simulink model "term"  (R2019b)
settings: Solver=VariableStepAuto  StartTime=0.0  StopTime=10  RelTol=1e-3
InitFcn:
  | clear all
  | given
values from neighbouring files (symbols this model uses):
  a0 = 0.01    [given.m]
  a1 = 1    [given.m]
  a2 = 1000    [given.m]
  a3 = 1000    [given.m]
  a4 = 10    [given.m]
  alpha = 0.9    [given.m]
  bar_B = [ ... (first row only)    [given.m]
  g = 9.81    [given.m]
  K = [-100 -100 -100 -10]    [given.m]
  kappa = 5    [given.m]
  N = 100    [given.m]
  psi0 = 0    [given.m]
  r0 = 5    [given.m]
  r1 = 10    [given.m]
  theta0 = 0    [given.m]
  x0 = 0    [given.m]
  y0 = 0    [given.m]
  z0 = 0    [given.m]
settings Model: Creator=bedla  LastModifiedBy=bedla

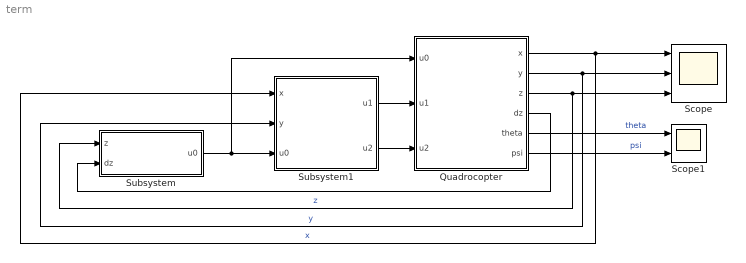
== system term ==
  Quadrocopter : Subsystem
  Scope : Scope  NumInputPorts=3
  Scope1 : Scope  NumInputPorts=2
  Subsystem : Subsystem
  Subsystem1 : Subsystem
  wires:
  Quadrocopter/3(z) -> Subsystem/1(z), Scope/3  "z"
  Subsystem1/1(u1) -> Quadrocopter/2(u1)
  Subsystem1/2(u2) -> Quadrocopter/3(u2)
  Quadrocopter/1(x) -> Subsystem1/1(x), Scope/1  "x"
  Quadrocopter/2(y) -> Subsystem1/2(y), Scope/2  "y"
  Quadrocopter/5(theta) -> Scope1/1  "theta"
  Quadrocopter/6(psi) -> Scope1/2  "psi"
  Subsystem/1(u0) -> Quadrocopter/1(u0), Subsystem1/3(u0)
  Quadrocopter/4(dz) -> Subsystem/2(dz)

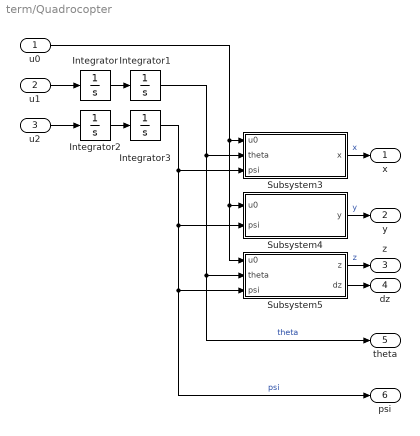
== system term/Quadrocopter ==
  u0 : Inport
  u1 : Inport  Port=2
  u2 : Inport  Port=3
  Integrator : Integrator
  Integrator1 : Integrator  InitialCondition=theta0
  Integrator2 : Integrator
  Integrator3 : Integrator  InitialCondition=psi0
  Subsystem3 : Subsystem
  Subsystem4 : Subsystem
  Subsystem5 : Subsystem
  x : Outport
  y : Outport  Port=2
  z : Outport  Port=3
  dz : Outport  Port=4
  theta : Outport  Port=5
  psi : Outport  Port=6
  wires:
  Integrator3/1 -> Subsystem3/3(psi), Subsystem4/2(psi), psi/1, Subsystem5/3(psi)  "psi"
  Integrator1/1 -> Subsystem3/2(theta), theta/1, Subsystem5/2(theta)  "theta"
  u0/1 -> Subsystem3/1(u0), Subsystem4/1(u0), Subsystem5/1(u0)
  Subsystem3/1(x) -> x/1  "x"
  Subsystem4/1(y) -> y/1  "y"
  Subsystem5/1(z) -> z/1  "z"
  Subsystem5/2(dz) -> dz/1
  u1/1 -> Integrator/1
  u2/1 -> Integrator2/1
  Integrator/1 -> Integrator1/1
  Integrator2/1 -> Integrator3/1

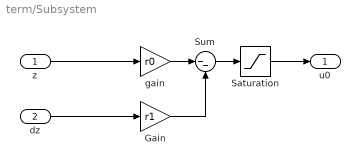
== system term/Subsystem ==
  z : Inport
  dz : Inport  Port=2
  Gain : Gain  Gain=r1
  Saturation : Saturate  UpperLimit=alpha*g  LowerLimit=-alpha*g
  Sum : Sum  Inputs=|--
  gain : Gain  Gain=r0
  u0 : Outport
  wires:
  Gain/1 -> Sum/2
  Saturation/1 -> u0/1
  z/1 -> gain/1
  gain/1 -> Sum/1
  dz/1 -> Gain/1
  Sum/1 -> Saturation/1

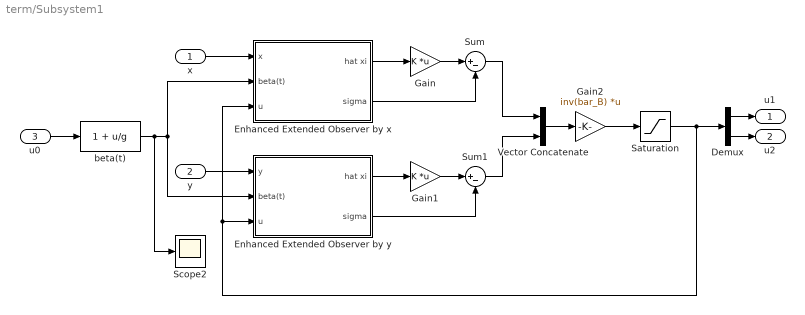
== system term/Subsystem1 ==
  x : Inport
  y : Inport  Port=2
  u0 : Inport  Port=3
  Demux : Demux  Outputs=2
  Enhanced Extended Observer by x : Subsystem
  Enhanced Extended Observer by y : Subsystem
  Gain : Gain  Gain=K  Multiplication=Matrix(K*u) (u vector)
  Gain1 : Gain  Gain=K  Multiplication=Matrix(K*u) (u vector)
  Gain2 : Gain  Gain=inv(bar_B)  Multiplication=Matrix(K*u) (u vector)
  Saturation : Saturate  UpperLimit=N  LowerLimit=-N
  Scope2 : Scope
  Sum : Sum  Inputs=|+-
  Sum1 : Sum  Inputs=|+-
  Vector Concatenate : Concatenate
  beta(t) : Fcn  Expr=1 + u/g
  u1 : Outport
  u2 : Outport  Port=2
  wires:
  Enhanced Extended Observer by x/1(hat xi) -> Gain/1
  Gain/1 -> Sum/1
  Enhanced Extended Observer by x/2(sigma) -> Sum/2
  Enhanced Extended Observer by y/2(sigma) -> Sum1/2
  Gain1/1 -> Sum1/1
  Enhanced Extended Observer by y/1(hat xi) -> Gain1/1
  Sum/1 -> Vector Concatenate/1
  Sum1/1 -> Vector Concatenate/2
  Vector Concatenate/1 -> Gain2/1
  Gain2/1 -> Saturation/1
  x/1 -> Enhanced Extended Observer by x/1(x)
  y/1 -> Enhanced Extended Observer by y/1(y)
  u0/1 -> beta(t)/1
  Demux/1 -> u1/1
  Demux/2 -> u2/1
  Saturation/1 -> Enhanced Extended Observer by x/3(u), Enhanced Extended Observer by y/3(u), Demux/1
  beta(t)/1 -> Scope2/1, Enhanced Extended Observer by y/2(beta(t)), Enhanced Extended Observer by x/2(beta(t))

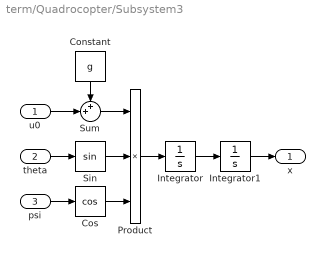
== system term/Quadrocopter/Subsystem3 ==
  u0 : Inport
  theta : Inport  Port=2
  psi : Inport  Port=3
  Constant : Constant  Value=g
  Cos : Trigonometry  Operator=cos
  Integrator : Integrator
  Integrator1 : Integrator  InitialCondition=x0
  Product : Product  Inputs=3
  Sin : Trigonometry
  Sum : Sum  Inputs=++|
  x : Outport
  wires:
  u0/1 -> Sum/2
  Cos/1 -> Product/3
  theta/1 -> Sin/1
  psi/1 -> Cos/1
  Sin/1 -> Product/2
  Product/1 -> Integrator/1
  Integrator/1 -> Integrator1/1
  Integrator1/1 -> x/1
  Sum/1 -> Product/1
  Constant/1 -> Sum/1

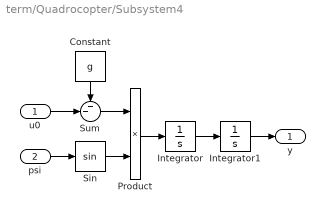
== system term/Quadrocopter/Subsystem4 ==
  u0 : Inport
  psi : Inport  Port=2
  Constant : Constant  Value=g
  Integrator : Integrator
  Integrator1 : Integrator  InitialCondition=y0
  Product : Product
  Sin : Trigonometry
  Sum : Sum  Inputs=--|
  y : Outport
  wires:
  Sin/1 -> Product/2
  psi/1 -> Sin/1
  Sum/1 -> Product/1
  u0/1 -> Sum/2
  Product/1 -> Integrator/1
  Integrator1/1 -> y/1
  Integrator/1 -> Integrator1/1
  Constant/1 -> Sum/1

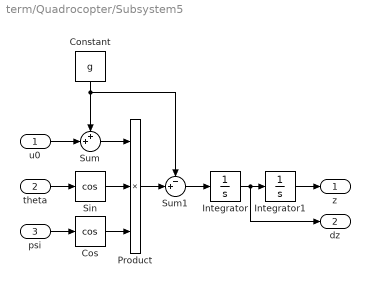
== system term/Quadrocopter/Subsystem5 ==
  u0 : Inport
  theta : Inport  Port=2
  psi : Inport  Port=3
  Constant : Constant  Value=g
  Cos : Trigonometry  Operator=cos
  Integrator : Integrator
  Integrator1 : Integrator  InitialCondition=z0
  Product : Product  Inputs=3
  Sin : Trigonometry  Operator=cos
  Sum : Sum  Inputs=++|
  Sum1 : Sum  Inputs=-+|
  z : Outport
  dz : Outport  Port=2
  wires:
  Sin/1 -> Product/2
  theta/1 -> Sin/1
  Constant/1 -> Sum1/1, Sum/1
  psi/1 -> Cos/1
  Integrator1/1 -> z/1
  Integrator/1 -> dz/1, Integrator1/1
  Cos/1 -> Product/3
  Product/1 -> Sum1/2
  Sum1/1 -> Integrator/1
  u0/1 -> Sum/2
  Sum/1 -> Product/1

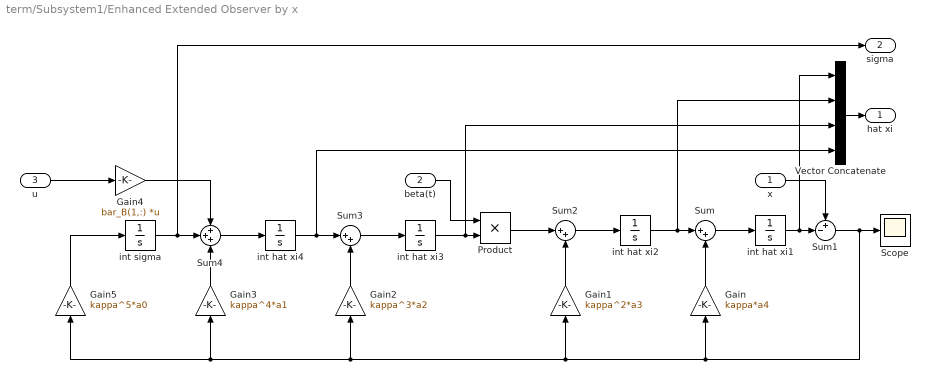
== system term/Subsystem1/Enhanced Extended Observer by x ==
  x : Inport
  beta(t) : Inport  Port=2
  u : Inport  Port=3
  Gain : Gain  Gain=kappa*a4
  Gain1 : Gain  Gain=kappa^2*a3
  Gain2 : Gain  Gain=kappa^3*a2
  Gain3 : Gain  Gain=kappa^4*a1
  Gain4 : Gain  Gain=bar_B(1,:)  Multiplication=Matrix(K*u) (u vector)
  Gain5 : Gain  Gain=kappa^5*a0
  Product : Product
  Scope : Scope
  Sum : Sum  Inputs=|++
  Sum1 : Sum  Inputs=+-|
  Sum2 : Sum  Inputs=|++
  Sum3 : Sum  Inputs=|++
  Sum4 : Sum  Inputs=+++
  Vector Concatenate : Concatenate  NumInputs=4
  int hat xi{1..4} (4 alike) : Integrator
  int sigma : Integrator
  hat xi : Outport
  sigma : Outport  Port=2
  wires:
  int hat xi2/1 -> Vector Concatenate/2, Sum/1
  Sum/1 -> int hat xi1/1
  int hat xi1/1 -> Vector Concatenate/1, Sum1/2
  x/1 -> Sum1/1
  Sum1/1 -> Scope/1, Gain/1, Gain5/1, Gain3/1, Gain2/1, Gain1/1
  Gain/1 -> Sum/2
  beta(t)/1 -> Product/1
  Product/1 -> Sum2/1
  Sum2/1 -> int hat xi2/1
  Gain1/1 -> Sum2/2
  Gain2/1 -> Sum3/2
  Sum3/1 -> int hat xi3/1
  int hat xi4/1 -> Vector Concatenate/4, Sum3/1
  Sum4/1 -> int hat xi4/1
  Gain3/1 -> Sum4/3
  int hat xi3/1 -> Vector Concatenate/3, Product/2
  int sigma/1 -> sigma/1, Sum4/2
  u/1 -> Gain4/1
  Gain5/1 -> int sigma/1
  Vector Concatenate/1 -> hat xi/1
  Gain4/1 -> Sum4/1

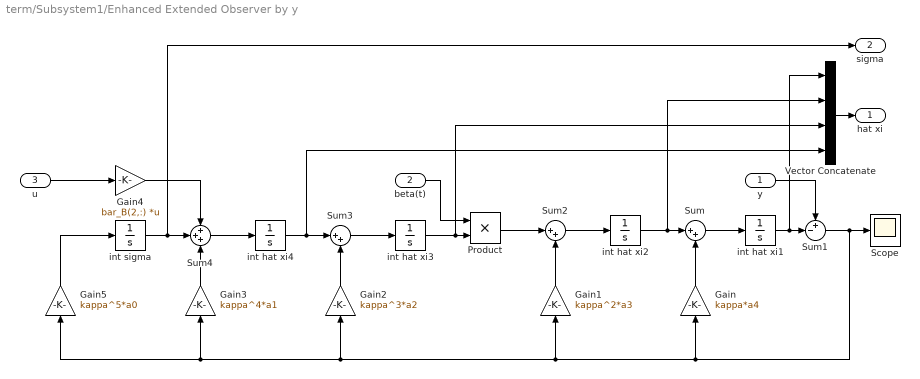
== system term/Subsystem1/Enhanced Extended Observer by y ==
  y : Inport
  beta(t) : Inport  Port=2
  u : Inport  Port=3
  Gain : Gain  Gain=kappa*a4
  Gain1 : Gain  Gain=kappa^2*a3
  Gain2 : Gain  Gain=kappa^3*a2
  Gain3 : Gain  Gain=kappa^4*a1
  Gain4 : Gain  Gain=bar_B(2,:)  Multiplication=Matrix(K*u) (u vector)
  Gain5 : Gain  Gain=kappa^5*a0
  Product : Product
  Scope : Scope
  Sum : Sum  Inputs=|++
  Sum1 : Sum  Inputs=+-|
  Sum2 : Sum  Inputs=|++
  Sum3 : Sum  Inputs=|++
  Sum4 : Sum  Inputs=+++
  Vector Concatenate : Concatenate  NumInputs=4
  int hat xi{1..4} (4 alike) : Integrator
  int sigma : Integrator
  hat xi : Outport
  sigma : Outport  Port=2
  wires:
  int hat xi2/1 -> Vector Concatenate/2, Sum/1
  Sum/1 -> int hat xi1/1
  int hat xi1/1 -> Vector Concatenate/1, Sum1/2
  y/1 -> Sum1/1
  Sum1/1 -> Scope/1, Gain/1, Gain5/1, Gain3/1, Gain2/1, Gain1/1
  Gain/1 -> Sum/2
  beta(t)/1 -> Product/1
  Product/1 -> Sum2/1
  Sum2/1 -> int hat xi2/1
  Gain1/1 -> Sum2/2
  Gain2/1 -> Sum3/2
  Sum3/1 -> int hat xi3/1
  int hat xi4/1 -> Vector Concatenate/4, Sum3/1
  Sum4/1 -> int hat xi4/1
  Gain3/1 -> Sum4/3
  int hat xi3/1 -> Vector Concatenate/3, Product/2
  int sigma/1 -> sigma/1, Sum4/2
  u/1 -> Gain4/1
  Gain5/1 -> int sigma/1
  Vector Concatenate/1 -> hat xi/1
  Gain4/1 -> Sum4/1
